simulink model "Simulation"  (R2024b)
settings: Solver=ode45  StartTime=0.0  StopTime=t_run  FixedStep=sim_time_step  RelTol=1e-6
values from neighbouring files (symbols this model uses):
  C = load("FeedbackController.mat")    [setupSimulationConfig.m]
undefined symbols (not defined in the file or in its folder): buffer_size, frequency_vector_1, frequency_vector_2, gain_vector_1, gain_vector_2, sim_time_step
libraries: slpidlib x4, cstblocks x3
settings Model: Creator=Ben  LastModifiedBy=Ben
settings ModelReferenceCC: EnableRefExpFcnMdlSchedulingChecks=on
settings RTWCC: GPUComputeCapability=3.5

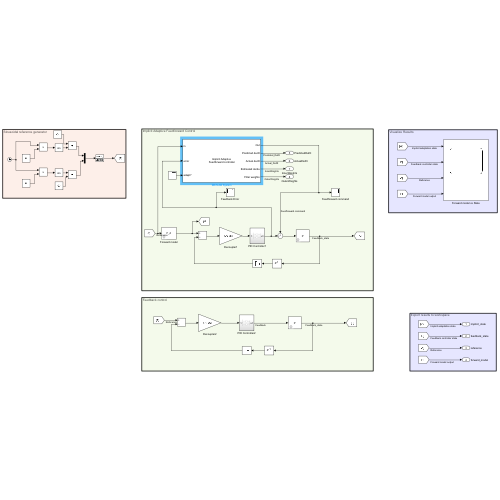
[thumbnail: Simulink's stored preview of the top-level diagram]
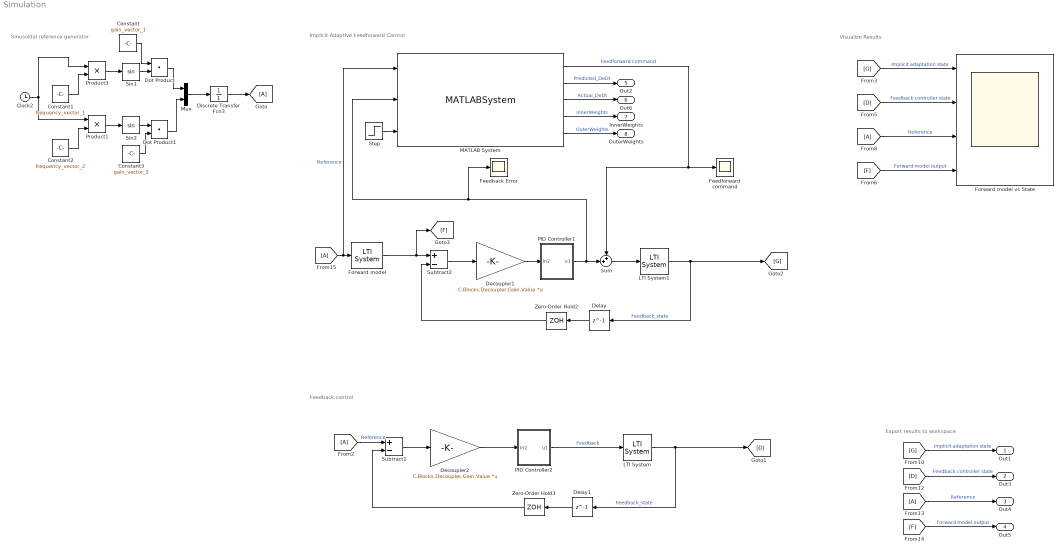
== system Simulation ==
  note: Export results to workspace
  note: Visualize Results
  note: Feedback control
  note: Sinusoidal reference generator
  note: Implicit Adaptive Feedforward Control
  Clock2 : Clock
  Constant : Constant  Value=gain_vector_1
  Constant1 : Constant  Value=frequency_vector_1
  Constant2 : Constant  Value=frequency_vector_2
  Constant3 : Constant  Value=gain_vector_2
  Decoupler1 : Gain  Gain=C.Blocks.Decoupler.Gain.Value  Multiplication=Matrix(K*u) (u vector)
  Decoupler2 : Gain  Gain=C.Blocks.Decoupler.Gain.Value  Multiplication=Matrix(K*u) (u vector)
  Delay : Delay  DelayLength=1
  Delay1 : Delay  DelayLength=1
  Discrete Transfer Fcn3 : DiscreteTransferFcn  Denominator=[1]  SampleTime=sim_time_step
  Dot Product : DotProduct  OutDataTypeStr=Inherit: Inherit via internal rule
  Dot Product1 : DotProduct  OutDataTypeStr=Inherit: Inherit via internal rule
  Feedback Error : Scope
  Feedforward command : Scope
  Forward model : cstblocks/LTI System  sys=F_d  IC=[]  PadeOrder=0
  Forward model vs State : Scope  NumInputPorts=4
  From{2,8,13,15} (4 alike) : From
  Goto : Goto
  LTI System : cstblocks/LTI System  sys=P  IC=[]  PadeOrder=0
  LTI System1 : cstblocks/LTI System  sys=P  IC=[]  PadeOrder=0
  MATLAB System : MATLABSystem  System=IAFF  alpha_gradient=alpha_gradient  alpha_reference=alpha_reference  L=buffer_size  N=2  M=2  K=2  SimulateUsing=Code generation  enableOutputDeDt=on  enableOutputDeDu=on  enableOutputWeights=on  variable_type=double  enableAdaptInput=on  initialWeightsScale=initialWeightsScale  initialWeightsSeed=initialWeightsSeed
      mask Type: IAFF
      mask Display:
      | disp(['Implicit Adaptive' char(10) ' Feedforward controller']);
      | port_label('input',1,'in');
      | port_label('input',2,'error');
      | port_label('input',3,'adapt?');
      | port_label('output',1,'Out');
      | port_label('output',2,'Predicted de/dt');
      | port_label('output',3,'Actual de/dt');
      | port_label('output',4,'Estimated de/du');
      | port_label('output',5,'Filter weights');
  Mux : Mux  Inputs=2
  PID Controller1 : Subsystem
  PID Controller2 : Subsystem
  Product1 : Product
  Product3 : Product
  Sin1 : Trigonometry
  Sin2 : Trigonometry
  Step : Step  Time=0  SampleTime=0
  Subtract1 : Sum  Inputs=+-
  Subtract2 : Sum  Inputs=+-
  Sum : Sum  Inputs=++|
  Zero-Order Hold2 : ZeroOrderHold  SampleTime=sim_time_step
  Zero-Order Hold3 : ZeroOrderHold  SampleTime=sim_time_step
  Out1 : Outport  SignalName=implicit_state
  Out3 : Outport  Port=2  SignalName=feedback_state
  Out4 : Outport  Port=3  SignalName=reference
  Out5 : Outport  Port=4  SignalName=forward_model
  Out2 : Outport  Port=5  SignalName=PredictedDeDt
  Out6 : Outport  Port=6  SignalName=ActualDeDt
  InnerWeights : Outport  Port=7
  OuterWeights : Outport  Port=8
  wires:
  [G] -> Forward model vs State/1  "Implicit adaptation state"
  [D] -> Forward model vs State/2  "Feedback controller state"
  [F] -> Forward model vs State/4  "Forward model output"
  From8/1 -> Forward model vs State/3  "Reference"
  [G] -> Out1/1  "Implicit adaptation state"
  [D] -> Out3/1  "Feedback controller state"
  From13/1 -> Out4/1  "Reference"
  [F] -> Out5/1  "Forward model output"
  Mux/1 -> Discrete Transfer Fcn3/1
  Discrete Transfer Fcn3/1 -> Goto/1
  PID Controller2/1(u1) -> LTI System/1  "Feedback"
  Decoupler2/1 -> PID Controller2/1(In2)
  From2/1 -> Subtract1/1  "Reference"
  Subtract1/1 -> Decoupler2/1
  LTI System/1 -> [D], Delay1/1  "Feedback_state"
  Decoupler1/1 -> PID Controller1/1(In2)
  Subtract2/1 -> Decoupler1/1
  From15/1 -> MATLAB System/1, Forward model/1  "Reference"
  LTI System1/1 -> [G], Delay/1  "Feedback_state"
  Constant1/1 -> Product3/2
  Product3/1 -> Sin1/1
  Constant2/1 -> Product1/2
  Clock2/1 -> Product3/1, Product1/1
  Product1/1 -> Sin2/1
  Sin1/1 -> Dot Product/2
  Dot Product/1 -> Mux/1
  Dot Product1/1 -> Mux/2
  Sin2/1 -> Dot Product1/1
  Constant/1 -> Dot Product/1
  Constant3/1 -> Dot Product1/2
  MATLAB System/1 -> Feedforward command/1, Sum/1  "Feedforward command"
  Zero-Order Hold2/1 -> Subtract2/2
  Zero-Order Hold3/1 -> Subtract1/2
  Forward model/1 -> [F], Subtract2/1
  Delay1/1 -> Zero-Order Hold3/1
  Delay/1 -> Zero-Order Hold2/1
  PID Controller1/1(u1) -> Feedback Error/1, MATLAB System/2, Sum/2
  Sum/1 -> LTI System1/1
  MATLAB System/3 -> Out6/1  "Actual_DeDt"
  MATLAB System/2 -> Out2/1  "Predicted_DeDt"
  MATLAB System/5 -> OuterWeights/1  "OuterWeights"
  MATLAB System/4 -> InnerWeights/1  "InnerWeights"
  Step/1 -> MATLAB System/3

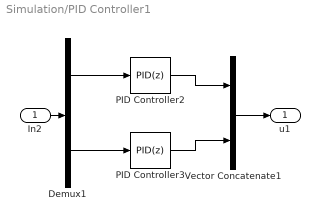
== system Simulation/PID Controller1 ==
  In2 : Inport
  Demux1 : Demux  Outputs=2
  PID Controller2 : slpidlib/PID Controller  Controller=PID  Form=Parallel  TimeDomain=Discrete-time  UseExternalTs=off  SampleTime=-1  IntegratorMethod=Forward Euler  FilterMethod=Forward Euler  ControllerParametersSource=internal  P=C.Blocks.PI_1.Kp.Value  I=C.Blocks.PI_1.Ki.Value  UseKiTs=off  D=C.Blocks.PI_1.Kd.Value  UseExternalDerivativeSource=off  N=C.Blocks.PI_1.Tf.Value  UseFilter=on  TunerSelectOption=Transfer Function Based (PID Tuner App)  InitialConditionSource=internal  InitialConditionForIntegrator=0  InitialConditionForFilter=0  DifferentiatorICPrevScaledInput=0  ExternalReset=none  TrackingMode=off  Kt=1  LimitOutput=off  SatLimitsSource=internal  UpperSaturationLimit=inf  LowerSaturationLimit=-inf  LinearizeAsGain=on  AntiWindupMode=none  Kb=1  LimitIntegrator=off  UpperIntegratorSaturationLimit=inf  LowerIntegratorSaturationLimit=-inf  POutMin=[]  POutMax=[]  IOutMin=[]  IOutMax=[]  DOutMin=[]  DOutMax=[]  NOutMin=[]  NOutMax=[]  SumOutMin=[]  SumOutMax=[]  SaturationOutMin=[]  SaturationOutMax=[]  PParamMin=[]  PParamMax=[]  IParamMin=[]  IParamMax=[]  DParamMin=[]  DParamMax=[]  NParamMin=[]  NParamMax=[]  KbParamMin=[]  KbParamMax=[]  KtParamMin=[]  KtParamMax=[]  KbOutMin=[]  KbOutMax=[]  KtOutMin=[]  KtOutMax=[]  IntegratorOutMin=[]  IntegratorOutMax=[]  FilterOutMin=[]  FilterOutMax=[]  SumI1OutMin=[]  SumI1OutMax=[]  SumI2OutMin=[]  SumI2OutMax=[]  SumI3OutMin=[]  SumI3OutMax=[]  SumI4OutMin=[]  SumI4OutMax=[]  SumDOutMin=[]  SumDOutMax=[]  DifferentiatorOutMin=[]  DifferentiatorOutMax=[]  FilterDiffOutCoefMin=[]  FilterDiffOutCoefMax=[]  ReciprocalOutMin=[]  ReciprocalOutMax=[]  SumDenOutMin=[]  SumDenOutMax=[]  SumNumOutMin=[]  SumNumOutMax=[]  DivideOutMin=[]  DivideOutMax=[]  UdiffTsProdOutMin=[]  UdiffTsProdOutMax=[]  NTsProdOutMin=[]  NTsProdOutMax=[]  UintegralTsProdOutMin=[]  UintegralTsProdOutMax=[]  UngainTsProdOutMin=[]  UngainTsProdOutMax=[]  ClampingZeroOutDataTypeStr=Inherit: Inherit via back propagation  ClampingZeroOutMin=[]  ClampingZeroOutMax=[]  FilterDenConstantOutDataTypeStr=Inherit: Inherit via back propagation  FilterDenConstantOutMin=[]  FilterDenConstantOutMax=[]  PCopyOutDataTypeStr=Inherit: Inherit via back propagation  PCopyOutMin=[]  PCopyOutMax=[]  NCopyOutDataTypeStr=Inherit: Inherit via back propagation  NCopyOutMin=[]  NCopyOutMax=[]  IntegratorContinuousStateAttributes=''  IntegratorStateMustResolveToSignalObject=off  IntegratorRTWStateStorageClass=Auto  FilterContinuousStateAttributes=''  FilterStateMustResolveToSignalObject=off  FilterRTWStateStorageClass=Auto  ParallelPVariant=InternalParameters  IdealPVariant=Disabled  IVariant=InternalParameters  DVariant=InternalParameters  IntegratorVariant=Discrete  SatVariant=Disabled  AWVariant=Passthrough  PCopyVariant=Disabled  TRVariant=Disabled  FdbkBlocksVariant=Forward  IdealPFdbkVariant=Disabled  SatFdbkVariant=Disabled  DerivativeFilterVariant=ForwardEulerFilter  NVariant=InternalParameters  NCopyVariant=Disabled  FilterICVariant=InternalICsFilter  IntegratorICVariant=InternalICs  ExternalResetVariant=Disabled  TRSumVariant=Passthrough  SumFdbkVariant=Disabled  SumVariant=Sum_PID  TsampFilterVariant=InternalTs  TsampNgainVariant=Passthrough  TsampIntegralVariant=Disabled_SignalSpec  ExternalSaturationOutDataTypeStr=Inherit: Same as second input  DerivativeSourceVariant=ErrorSignal  PreIntVariant=InternalPreInt
  PID Controller3 : slpidlib/PID Controller  Controller=PID  Form=Parallel  TimeDomain=Discrete-time  UseExternalTs=off  SampleTime=-1  IntegratorMethod=Forward Euler  FilterMethod=Forward Euler  ControllerParametersSource=internal  P=C.Blocks.PI_2.Kp.Value  I=C.Blocks.PI_2.Ki.Value  UseKiTs=off  D=C.Blocks.PI_2.Kd.Value  UseExternalDerivativeSource=off  N=C.Blocks.PI_2.Tf.Value  UseFilter=on  TunerSelectOption=Transfer Function Based (PID Tuner App)  InitialConditionSource=internal  InitialConditionForIntegrator=0  InitialConditionForFilter=0  DifferentiatorICPrevScaledInput=0  ExternalReset=none  TrackingMode=off  Kt=1  LimitOutput=off  SatLimitsSource=internal  UpperSaturationLimit=inf  LowerSaturationLimit=-inf  LinearizeAsGain=on  AntiWindupMode=none  Kb=1  LimitIntegrator=off  UpperIntegratorSaturationLimit=inf  LowerIntegratorSaturationLimit=-inf  POutMin=[]  POutMax=[]  IOutMin=[]  IOutMax=[]  DOutMin=[]  DOutMax=[]  NOutMin=[]  NOutMax=[]  SumOutMin=[]  SumOutMax=[]  SaturationOutMin=[]  SaturationOutMax=[]  PParamMin=[]  PParamMax=[]  IParamMin=[]  IParamMax=[]  DParamMin=[]  DParamMax=[]  NParamMin=[]  NParamMax=[]  KbParamMin=[]  KbParamMax=[]  KtParamMin=[]  KtParamMax=[]  KbOutMin=[]  KbOutMax=[]  KtOutMin=[]  KtOutMax=[]  IntegratorOutMin=[]  IntegratorOutMax=[]  FilterOutMin=[]  FilterOutMax=[]  SumI1OutMin=[]  SumI1OutMax=[]  SumI2OutMin=[]  SumI2OutMax=[]  SumI3OutMin=[]  SumI3OutMax=[]  SumI4OutMin=[]  SumI4OutMax=[]  SumDOutMin=[]  SumDOutMax=[]  DifferentiatorOutMin=[]  DifferentiatorOutMax=[]  FilterDiffOutCoefMin=[]  FilterDiffOutCoefMax=[]  ReciprocalOutMin=[]  ReciprocalOutMax=[]  SumDenOutMin=[]  SumDenOutMax=[]  SumNumOutMin=[]  SumNumOutMax=[]  DivideOutMin=[]  DivideOutMax=[]  UdiffTsProdOutMin=[]  UdiffTsProdOutMax=[]  NTsProdOutMin=[]  NTsProdOutMax=[]  UintegralTsProdOutMin=[]  UintegralTsProdOutMax=[]  UngainTsProdOutMin=[]  UngainTsProdOutMax=[]  ClampingZeroOutDataTypeStr=Inherit: Inherit via back propagation  ClampingZeroOutMin=[]  ClampingZeroOutMax=[]  FilterDenConstantOutDataTypeStr=Inherit: Inherit via back propagation  FilterDenConstantOutMin=[]  FilterDenConstantOutMax=[]  PCopyOutDataTypeStr=Inherit: Inherit via back propagation  PCopyOutMin=[]  PCopyOutMax=[]  NCopyOutDataTypeStr=Inherit: Inherit via back propagation  NCopyOutMin=[]  NCopyOutMax=[]  IntegratorContinuousStateAttributes=''  IntegratorStateMustResolveToSignalObject=off  IntegratorRTWStateStorageClass=Auto  FilterContinuousStateAttributes=''  FilterStateMustResolveToSignalObject=off  FilterRTWStateStorageClass=Auto  ParallelPVariant=InternalParameters  IdealPVariant=Disabled  IVariant=InternalParameters  DVariant=InternalParameters  IntegratorVariant=Discrete  SatVariant=Disabled  AWVariant=Passthrough  PCopyVariant=Disabled  TRVariant=Disabled  FdbkBlocksVariant=Forward  IdealPFdbkVariant=Disabled  SatFdbkVariant=Disabled  DerivativeFilterVariant=ForwardEulerFilter  NVariant=InternalParameters  NCopyVariant=Disabled  FilterICVariant=InternalICsFilter  IntegratorICVariant=InternalICs  ExternalResetVariant=Disabled  TRSumVariant=Passthrough  SumFdbkVariant=Disabled  SumVariant=Sum_PID  TsampFilterVariant=InternalTs  TsampNgainVariant=Passthrough  TsampIntegralVariant=Disabled_SignalSpec  ExternalSaturationOutDataTypeStr=Inherit: Same as second input  DerivativeSourceVariant=ErrorSignal  PreIntVariant=InternalPreInt
  Vector Concatenate1 : Concatenate
  u1 : Outport
  wires:
  In2/1 -> Demux1/1
  PID Controller2/1 -> Vector Concatenate1/1
  PID Controller3/1 -> Vector Concatenate1/2
  Vector Concatenate1/1 -> u1/1
  Demux1/1 -> PID Controller2/1
  Demux1/2 -> PID Controller3/1

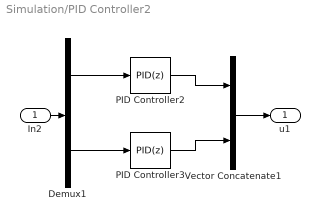
== system Simulation/PID Controller2 ==
  In2 : Inport
  Demux1 : Demux  Outputs=2
  PID Controller2 : slpidlib/PID Controller  Controller=PID  Form=Parallel  TimeDomain=Discrete-time  UseExternalTs=off  SampleTime=-1  IntegratorMethod=Forward Euler  FilterMethod=Forward Euler  ControllerParametersSource=internal  P=C.Blocks.PI_1.Kp.Value  I=C.Blocks.PI_1.Ki.Value  UseKiTs=off  D=C.Blocks.PI_1.Kd.Value  UseExternalDerivativeSource=off  N=C.Blocks.PI_1.Tf.Value  UseFilter=on  TunerSelectOption=Transfer Function Based (PID Tuner App)  InitialConditionSource=internal  InitialConditionForIntegrator=0  InitialConditionForFilter=0  DifferentiatorICPrevScaledInput=0  ExternalReset=none  TrackingMode=off  Kt=1  LimitOutput=off  SatLimitsSource=internal  UpperSaturationLimit=inf  LowerSaturationLimit=-inf  LinearizeAsGain=on  AntiWindupMode=none  Kb=1  LimitIntegrator=off  UpperIntegratorSaturationLimit=inf  LowerIntegratorSaturationLimit=-inf  POutMin=[]  POutMax=[]  IOutMin=[]  IOutMax=[]  DOutMin=[]  DOutMax=[]  NOutMin=[]  NOutMax=[]  SumOutMin=[]  SumOutMax=[]  SaturationOutMin=[]  SaturationOutMax=[]  PParamMin=[]  PParamMax=[]  IParamMin=[]  IParamMax=[]  DParamMin=[]  DParamMax=[]  NParamMin=[]  NParamMax=[]  KbParamMin=[]  KbParamMax=[]  KtParamMin=[]  KtParamMax=[]  KbOutMin=[]  KbOutMax=[]  KtOutMin=[]  KtOutMax=[]  IntegratorOutMin=[]  IntegratorOutMax=[]  FilterOutMin=[]  FilterOutMax=[]  SumI1OutMin=[]  SumI1OutMax=[]  SumI2OutMin=[]  SumI2OutMax=[]  SumI3OutMin=[]  SumI3OutMax=[]  SumI4OutMin=[]  SumI4OutMax=[]  SumDOutMin=[]  SumDOutMax=[]  DifferentiatorOutMin=[]  DifferentiatorOutMax=[]  FilterDiffOutCoefMin=[]  FilterDiffOutCoefMax=[]  ReciprocalOutMin=[]  ReciprocalOutMax=[]  SumDenOutMin=[]  SumDenOutMax=[]  SumNumOutMin=[]  SumNumOutMax=[]  DivideOutMin=[]  DivideOutMax=[]  UdiffTsProdOutMin=[]  UdiffTsProdOutMax=[]  NTsProdOutMin=[]  NTsProdOutMax=[]  UintegralTsProdOutMin=[]  UintegralTsProdOutMax=[]  UngainTsProdOutMin=[]  UngainTsProdOutMax=[]  ClampingZeroOutDataTypeStr=Inherit: Inherit via back propagation  ClampingZeroOutMin=[]  ClampingZeroOutMax=[]  FilterDenConstantOutDataTypeStr=Inherit: Inherit via back propagation  FilterDenConstantOutMin=[]  FilterDenConstantOutMax=[]  PCopyOutDataTypeStr=Inherit: Inherit via back propagation  PCopyOutMin=[]  PCopyOutMax=[]  NCopyOutDataTypeStr=Inherit: Inherit via back propagation  NCopyOutMin=[]  NCopyOutMax=[]  IntegratorContinuousStateAttributes=''  IntegratorStateMustResolveToSignalObject=off  IntegratorRTWStateStorageClass=Auto  FilterContinuousStateAttributes=''  FilterStateMustResolveToSignalObject=off  FilterRTWStateStorageClass=Auto  ParallelPVariant=InternalParameters  IdealPVariant=Disabled  IVariant=InternalParameters  DVariant=InternalParameters  IntegratorVariant=Discrete  SatVariant=Disabled  AWVariant=Passthrough  PCopyVariant=Disabled  TRVariant=Disabled  FdbkBlocksVariant=Forward  IdealPFdbkVariant=Disabled  SatFdbkVariant=Disabled  DerivativeFilterVariant=ForwardEulerFilter  NVariant=InternalParameters  NCopyVariant=Disabled  FilterICVariant=InternalICsFilter  IntegratorICVariant=InternalICs  ExternalResetVariant=Disabled  TRSumVariant=Passthrough  SumFdbkVariant=Disabled  SumVariant=Sum_PID  TsampFilterVariant=InternalTs  TsampNgainVariant=Passthrough  TsampIntegralVariant=Disabled_SignalSpec  ExternalSaturationOutDataTypeStr=Inherit: Same as second input  DerivativeSourceVariant=ErrorSignal  PreIntVariant=InternalPreInt
  PID Controller3 : slpidlib/PID Controller  Controller=PID  Form=Parallel  TimeDomain=Discrete-time  UseExternalTs=off  SampleTime=-1  IntegratorMethod=Forward Euler  FilterMethod=Forward Euler  ControllerParametersSource=internal  P=C.Blocks.PI_2.Kp.Value  I=C.Blocks.PI_2.Ki.Value  UseKiTs=off  D=C.Blocks.PI_2.Kd.Value  UseExternalDerivativeSource=off  N=C.Blocks.PI_2.Tf.Value  UseFilter=on  TunerSelectOption=Transfer Function Based (PID Tuner App)  InitialConditionSource=internal  InitialConditionForIntegrator=0  InitialConditionForFilter=0  DifferentiatorICPrevScaledInput=0  ExternalReset=none  TrackingMode=off  Kt=1  LimitOutput=off  SatLimitsSource=internal  UpperSaturationLimit=inf  LowerSaturationLimit=-inf  LinearizeAsGain=on  AntiWindupMode=none  Kb=1  LimitIntegrator=off  UpperIntegratorSaturationLimit=inf  LowerIntegratorSaturationLimit=-inf  POutMin=[]  POutMax=[]  IOutMin=[]  IOutMax=[]  DOutMin=[]  DOutMax=[]  NOutMin=[]  NOutMax=[]  SumOutMin=[]  SumOutMax=[]  SaturationOutMin=[]  SaturationOutMax=[]  PParamMin=[]  PParamMax=[]  IParamMin=[]  IParamMax=[]  DParamMin=[]  DParamMax=[]  NParamMin=[]  NParamMax=[]  KbParamMin=[]  KbParamMax=[]  KtParamMin=[]  KtParamMax=[]  KbOutMin=[]  KbOutMax=[]  KtOutMin=[]  KtOutMax=[]  IntegratorOutMin=[]  IntegratorOutMax=[]  FilterOutMin=[]  FilterOutMax=[]  SumI1OutMin=[]  SumI1OutMax=[]  SumI2OutMin=[]  SumI2OutMax=[]  SumI3OutMin=[]  SumI3OutMax=[]  SumI4OutMin=[]  SumI4OutMax=[]  SumDOutMin=[]  SumDOutMax=[]  DifferentiatorOutMin=[]  DifferentiatorOutMax=[]  FilterDiffOutCoefMin=[]  FilterDiffOutCoefMax=[]  ReciprocalOutMin=[]  ReciprocalOutMax=[]  SumDenOutMin=[]  SumDenOutMax=[]  SumNumOutMin=[]  SumNumOutMax=[]  DivideOutMin=[]  DivideOutMax=[]  UdiffTsProdOutMin=[]  UdiffTsProdOutMax=[]  NTsProdOutMin=[]  NTsProdOutMax=[]  UintegralTsProdOutMin=[]  UintegralTsProdOutMax=[]  UngainTsProdOutMin=[]  UngainTsProdOutMax=[]  ClampingZeroOutDataTypeStr=Inherit: Inherit via back propagation  ClampingZeroOutMin=[]  ClampingZeroOutMax=[]  FilterDenConstantOutDataTypeStr=Inherit: Inherit via back propagation  FilterDenConstantOutMin=[]  FilterDenConstantOutMax=[]  PCopyOutDataTypeStr=Inherit: Inherit via back propagation  PCopyOutMin=[]  PCopyOutMax=[]  NCopyOutDataTypeStr=Inherit: Inherit via back propagation  NCopyOutMin=[]  NCopyOutMax=[]  IntegratorContinuousStateAttributes=''  IntegratorStateMustResolveToSignalObject=off  IntegratorRTWStateStorageClass=Auto  FilterContinuousStateAttributes=''  FilterStateMustResolveToSignalObject=off  FilterRTWStateStorageClass=Auto  ParallelPVariant=InternalParameters  IdealPVariant=Disabled  IVariant=InternalParameters  DVariant=InternalParameters  IntegratorVariant=Discrete  SatVariant=Disabled  AWVariant=Passthrough  PCopyVariant=Disabled  TRVariant=Disabled  FdbkBlocksVariant=Forward  IdealPFdbkVariant=Disabled  SatFdbkVariant=Disabled  DerivativeFilterVariant=ForwardEulerFilter  NVariant=InternalParameters  NCopyVariant=Disabled  FilterICVariant=InternalICsFilter  IntegratorICVariant=InternalICs  ExternalResetVariant=Disabled  TRSumVariant=Passthrough  SumFdbkVariant=Disabled  SumVariant=Sum_PID  TsampFilterVariant=InternalTs  TsampNgainVariant=Passthrough  TsampIntegralVariant=Disabled_SignalSpec  ExternalSaturationOutDataTypeStr=Inherit: Same as second input  DerivativeSourceVariant=ErrorSignal  PreIntVariant=InternalPreInt
  Vector Concatenate1 : Concatenate
  u1 : Outport
  wires:
  In2/1 -> Demux1/1
  PID Controller2/1 -> Vector Concatenate1/1
  PID Controller3/1 -> Vector Concatenate1/2
  Vector Concatenate1/1 -> u1/1
  Demux1/1 -> PID Controller2/1
  Demux1/2 -> PID Controller3/1
